simulink model "dynamique_vehicle"  (R2018a)
settings: Solver=ode45  StartTime=0.0  StopTime=10.0  RelTol=1e-3
values from neighbouring files (symbols this model uses):
  Dpitch_h = 1    [Constante.m]
  Droll = hg - (h2+ L2*sin(atan((h1+h2)/L)))    [Constante.m]
  DrollF = DshockF*E1^2    (= 1.44)    [Constante.m]
  DrollR = DshockR*E2^2    (= 1.44)    [Constante.m]
  g = 9.81    [Constante.m]
  Itotx = 1    [Constante.m]
  Itoty = 1    [Constante.m]
  Kpitch_h = 1    [Constante.m]
  KrollF = KspringF*E1^2/2 + KantirollF    (= 1.72)    [Constante.m]
  KrollR = KspringR*E2^2/2 + KantirollR    (= 1.72)    [Constante.m]
  Mtot = 220    [Constante.m]
  Vx0 = 0    [Constante.m]
  Vy0 = 0    [Constante.m]
  Wz0 = 0    [Constante.m]
  X0 = 0    [Constante.m]
  Y0 = 0    [Constante.m]
  yaw0 = 0    [Constante.m]
undefined symbols (not defined in the file or in its folder): Fx1, Fx2, Fx3, Fx4, Fy1, Fy2, Fy3, Fy4
libraries: autolibshareddiff x1
settings Model: Creator=bobau  LastModifiedBy=bobau

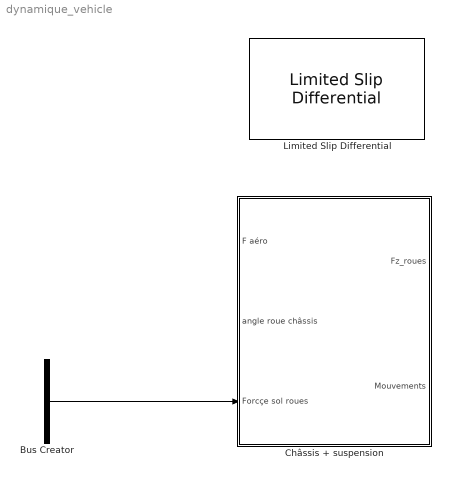
== system dynamique_vehicle ==
  Bus Creator : BusCreator  Inputs=Fy1,Fx1,Fy2,Fx2,Fy3,Fx3,Fy4,Fx4
  Châssis + suspension : Subsystem
  Limited Slip Differential : autolibshareddiff/Limited Slip Differential  shaftSwitchMask=To the left of center-line  Ndiff=4  Jd=.1  bd=1e-3  Jw1=.1  bw1=1e-3  Jw2=.1  bw2=1e-3  omegaw1o=0  omegaw2o=0  couplingType=Pre-loaded ideal clutch  Ndisks=4  Reff=.20  Fc=500  muc=[.16 0.13 0.115 0.11 0.105 0.1025 0.10125]  dw=[0 10 20 40 60 80 100]  Tdw=[-100, -90, -50, -5, 0, 5, 50, 90, 100]  dwT=[-200, -175, -100, - 50, 0, 50, 100, 175, 200]  TTin=[-200 -175 -100 - 50 0 50 100 175 200]  Tin=[-200 -175 -100 - 50 0 50 100 175 200]  tauC=.01  IdealInterpMethod=Linear  IdealExtrapMethod=Clip  TdwInterpMethod=Linear  TdwExtrapMethod=Clip  TTinInterpMethod=Linear  TTinExtrapMethod=Clip  maxAbsSpd=5e3  aMode=2
      settings: SourceProductName=Powertrain Blockset  SourceProductBaseCode=PW
  wires:
  Bus Creator/1 -> Châssis + suspension/3(Forcçe sol roues)

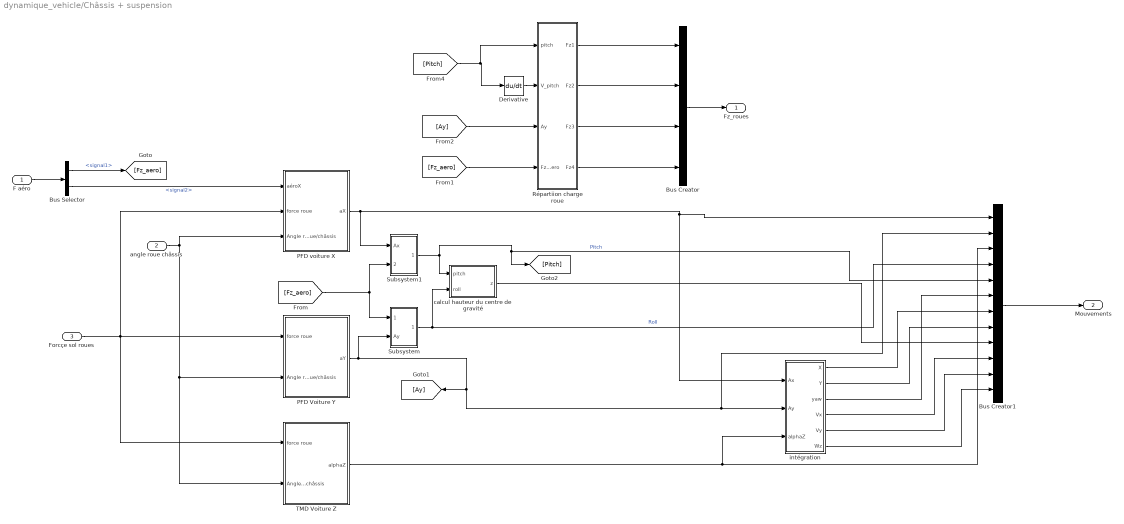
== system dynamique_vehicle/Châssis + suspension ==
  F aéro : Inport
  angle roue châssis : Inport  Port=2
  Forcçe sol roues : Inport  Port=3
  Bus Creator : BusCreator  Inputs=4
  Bus Creator1 : BusCreator  Inputs=12
  Bus Selector : BusSelector  OutputSignals=signal1,signal2
  Derivative : Derivative
  PFD Voiture Y : Subsystem
  PFD voiture X : Subsystem
  Répartiion charge roue : MATLAB Function  TreatAsAtomicUnit=on
  Subsystem : Subsystem
  Subsystem1 : Subsystem
  TMD Voiture Z : Subsystem
  calcul hauteur du centre de gravité : MATLAB Function  TreatAsAtomicUnit=on
  intégration : Subsystem
  Fz_roues : Outport
  Mouvements : Outport  Port=2
  wires:
  Forcçe sol roues/1 -> PFD Voiture Y/1("force roue "), TMD Voiture Z/1("force roue "), PFD voiture X/2("force roue ")
  angle roue châssis/1 -> PFD Voiture Y/2(Angle roue/châssis), TMD Voiture Z/2(Angle roue/châssis), PFD voiture X/3(Angle roue/châssis)
  PFD voiture X/1(aX) -> Bus Creator1/1, intégration/1(Ax), Subsystem1/1(Ax)
  Subsystem/1(Roll) -> calcul hauteur du centre de gravité/2(roll), Bus Creator1/4  "Roll"
  PFD Voiture Y/1(aY) -> Subsystem/2(Ay), Bus Creator1/2, intégration/2(Ay), [Ay]
  Subsystem1/1(Pitch) -> Bus Creator1/5, [Pitch], calcul hauteur du centre de gravité/1(pitch)  "Pitch"
  calcul hauteur du centre de gravité/1(z) -> Bus Creator1/9
  F aéro/1 -> Bus Selector/1
  Bus Selector/2 -> PFD voiture X/1(aéroX)  "<signal2>"
  Bus Selector/1 -> [Fz_aero]  "<signal1>"
  [Fz_aero] -> Subsystem1/2(Fz aéro), Subsystem/1(Fy aéro)
  Derivative/1 -> Répartiion charge roue/2(V_pitch)
  [Fz_aero] -> Répartiion charge roue/4(Fz_aero)
  [Pitch] -> Répartiion charge roue/1(pitch), Derivative/1
  [Ay] -> Répartiion charge roue/3(Ay)
  Répartiion charge roue/1(Fz1) -> Bus Creator/1
  Répartiion charge roue/4(Fz4) -> Bus Creator/4
  Répartiion charge roue/3(Fz3) -> Bus Creator/3
  Répartiion charge roue/2(Fz2) -> Bus Creator/2
  Bus Creator/1 -> Fz_roues/1
  Bus Creator1/1 -> Mouvements/1
  TMD Voiture Z/1(alphaZ) -> Bus Creator1/3, intégration/3(alphaZ)
  intégration/6(Wz) -> Bus Creator1/12
  intégration/5(Vy) -> Bus Creator1/11
  intégration/4(Vx) -> Bus Creator1/10
  intégration/3(yaw) -> Bus Creator1/6
  intégration/2(Y) -> Bus Creator1/8
  intégration/1(X) -> Bus Creator1/7

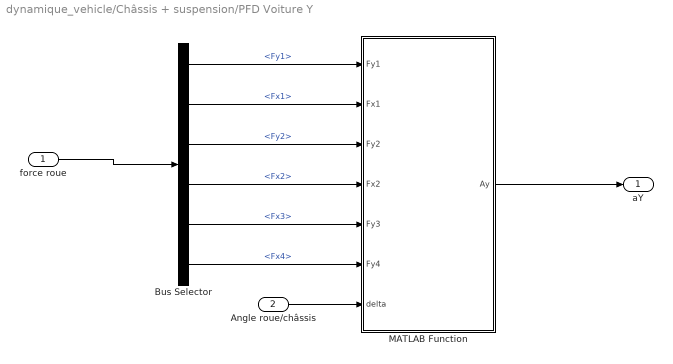
== system dynamique_vehicle/Châssis + suspension/PFD Voiture Y ==
  "force roue " : Inport
  Angle roue/châssis : Inport  Port=2
  Bus Selector : BusSelector  OutputSignals=Fy1,Fx1,Fy2,Fx2,Fx3,Fx4
  MATLAB Function : MATLAB Function  TreatAsAtomicUnit=on
  aY : Outport
  wires:
  Bus Selector/5 -> MATLAB Function/5(Fy3)  "<Fx3>"
  Bus Selector/4 -> MATLAB Function/4(Fx2)  "<Fx2>"
  Bus Selector/3 -> MATLAB Function/3(Fy2)  "<Fy2>"
  Bus Selector/2 -> MATLAB Function/2(Fx1)  "<Fx1>"
  Bus Selector/1 -> MATLAB Function/1(Fy1)  "<Fy1>"
  Bus Selector/6 -> MATLAB Function/6(Fy4)  "<Fx4>"
  Angle roue/châssis/1 -> MATLAB Function/7(delta)
  MATLAB Function/1(Ay) -> aY/1
  "force roue "/1 -> Bus Selector/1

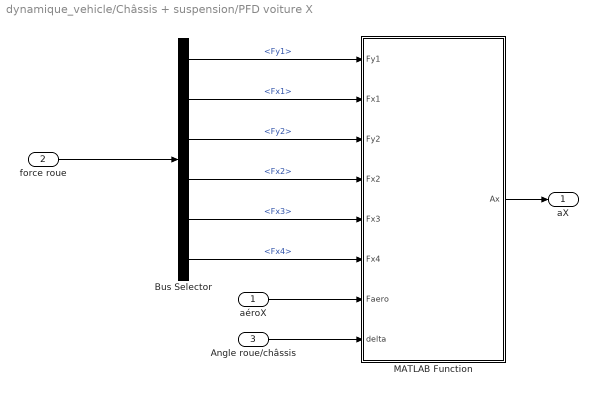
== system dynamique_vehicle/Châssis + suspension/PFD voiture X ==
  aéroX : Inport
  "force roue " : Inport  Port=2
  Angle roue/châssis : Inport  Port=3
  Bus Selector : BusSelector  OutputSignals=Fy1,Fx1,Fy2,Fx2,Fx3,Fx4
  MATLAB Function : MATLAB Function  TreatAsAtomicUnit=on
  aX : Outport
  wires:
  "force roue "/1 -> Bus Selector/1
  MATLAB Function/1(Ax) -> aX/1
  Angle roue/châssis/1 -> MATLAB Function/8(delta)
  Bus Selector/6 -> MATLAB Function/6(Fx4)  "<Fx4>"
  Bus Selector/1 -> MATLAB Function/1(Fy1)  "<Fy1>"
  Bus Selector/2 -> MATLAB Function/2(Fx1)  "<Fx1>"
  Bus Selector/3 -> MATLAB Function/3(Fy2)  "<Fy2>"
  Bus Selector/4 -> MATLAB Function/4(Fx2)  "<Fx2>"
  Bus Selector/5 -> MATLAB Function/5(Fx3)  "<Fx3>"
  aéroX/1 -> MATLAB Function/7(Faero)

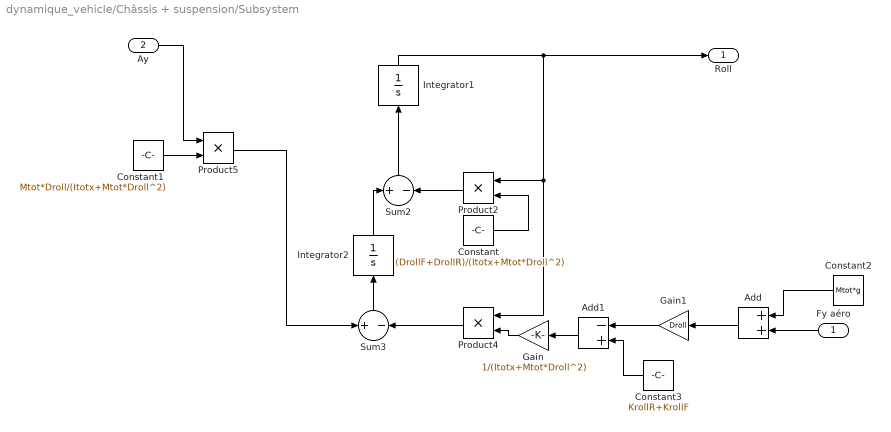
== system dynamique_vehicle/Châssis + suspension/Subsystem ==
  Fy aéro : Inport
  Ay : Inport  Port=2
  Add : Sum
  Add1 : Sum  Inputs=-+
  Constant : Constant  Value=(DrollF+DrollR)/(Itotx+Mtot*Droll^2)
  Constant1 : Constant  Value=Mtot*Droll/(Itotx+Mtot*Droll^2)
  Constant2 : Constant  Value=Mtot*g
  Constant3 : Constant  Value=KrollR+KrollF
  Gain : Gain  Gain=1/(Itotx+Mtot*Droll^2)
  Gain1 : Gain  Gain=Droll
  Integrator1 : Integrator
  Integrator2 : Integrator
  Product2 : Product  SaturateOnIntegerOverflow=on  RndMeth=Zero  InputSameDT=on  OutDataTypeStr=Inherit: Same as first input
  Product4 : Product  SaturateOnIntegerOverflow=on  RndMeth=Zero  InputSameDT=on  OutDataTypeStr=Inherit: Same as first input
  Product5 : Product  SaturateOnIntegerOverflow=on  RndMeth=Zero  InputSameDT=on  OutDataTypeStr=Inherit: Same as first input
  Sum2 : Sum  Inputs=+|-  SaturateOnIntegerOverflow=on  InputSameDT=on  OutDataTypeStr=Inherit: Same as first input
  Sum3 : Sum  Inputs=+|-  SaturateOnIntegerOverflow=on  InputSameDT=on  OutDataTypeStr=Inherit: Same as first input
  Roll : Outport
  wires:
  Ay/1 -> Product5/1
  Product2/1 -> Sum2/2
  Constant/1 -> Product2/2
  Sum3/1 -> Integrator2/1
  Sum2/1 -> Integrator1/1
  Integrator1/1 -> Roll/1, Product2/1, Product4/1
  Gain/1 -> Product4/2
  Product4/1 -> Sum3/2
  Constant3/1 -> Add1/2
  Integrator2/1 -> Sum2/1
  Product5/1 -> Sum3/1
  Constant2/1 -> Add/1
  Add1/1 -> Gain/1
  Constant1/1 -> Product5/2
  Fy aéro/1 -> Add/2
  Gain1/1 -> Add1/1
  Add/1 -> Gain1/1

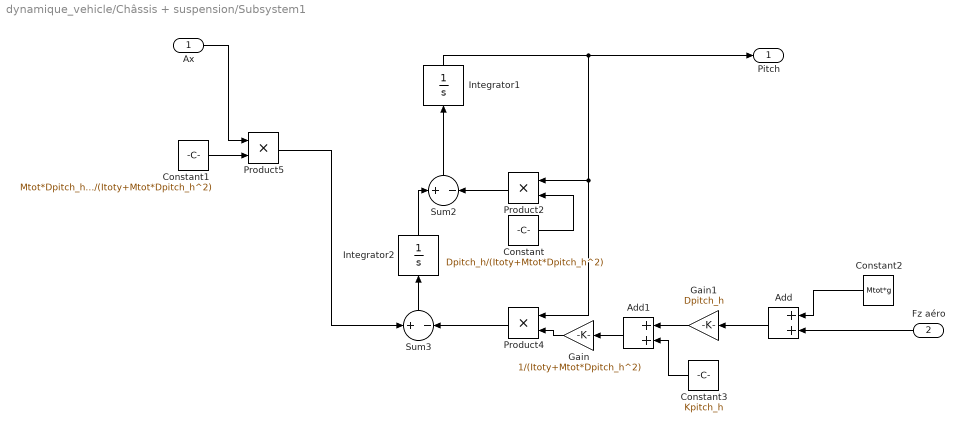
== system dynamique_vehicle/Châssis + suspension/Subsystem1 ==
  Ax : Inport
  Fz aéro : Inport  Port=2
  Add : Sum
  Add1 : Sum
  Constant : Constant  Value=Dpitch_h/(Itoty+Mtot*Dpitch_h^2)
  Constant1 : Constant  Value=Mtot*Dpitch_h/(Itoty+Mtot*Dpitch_h^2)
  Constant2 : Constant  Value=Mtot*g
  Constant3 : Constant  Value=Kpitch_h
  Gain : Gain  Gain=1/(Itoty+Mtot*Dpitch_h^2)
  Gain1 : Gain  Gain=Dpitch_h
  Integrator1 : Integrator
  Integrator2 : Integrator
  Product2 : Product  SaturateOnIntegerOverflow=on  RndMeth=Zero  InputSameDT=on  OutDataTypeStr=Inherit: Same as first input
  Product4 : Product  SaturateOnIntegerOverflow=on  RndMeth=Zero  InputSameDT=on  OutDataTypeStr=Inherit: Same as first input
  Product5 : Product  SaturateOnIntegerOverflow=on  RndMeth=Zero  InputSameDT=on  OutDataTypeStr=Inherit: Same as first input
  Sum2 : Sum  Inputs=+|-  SaturateOnIntegerOverflow=on  InputSameDT=on  OutDataTypeStr=Inherit: Same as first input
  Sum3 : Sum  Inputs=+|-  SaturateOnIntegerOverflow=on  InputSameDT=on  OutDataTypeStr=Inherit: Same as first input
  Pitch : Outport
  wires:
  Fz aéro/1 -> Add/2
  Constant1/1 -> Product5/2
  Add1/1 -> Gain/1
  Constant2/1 -> Add/1
  Product5/1 -> Sum3/1
  Integrator2/1 -> Sum2/1
  Constant3/1 -> Add1/2
  Product4/1 -> Sum3/2
  Gain/1 -> Product4/2
  Integrator1/1 -> Product4/1, Product2/1, Pitch/1
  Sum2/1 -> Integrator1/1
  Sum3/1 -> Integrator2/1
  Constant/1 -> Product2/2
  Product2/1 -> Sum2/2
  Ax/1 -> Product5/1
  Add/1 -> Gain1/1
  Gain1/1 -> Add1/1

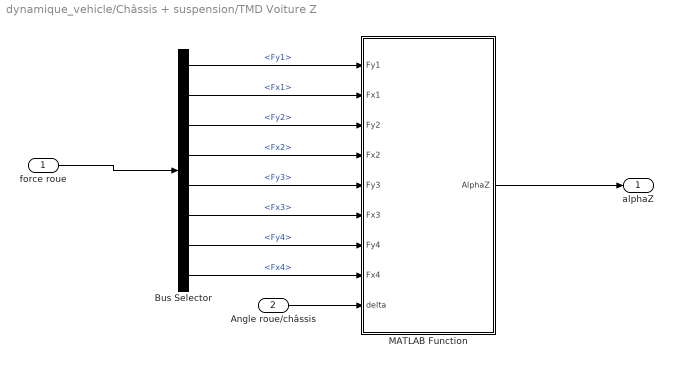
== system dynamique_vehicle/Châssis + suspension/TMD Voiture Z ==
  "force roue " : Inport
  Angle roue/châssis : Inport  Port=2
  Bus Selector : BusSelector  OutputSignals=Fy1,Fx1,Fy2,Fx2,Fy3,Fx3,Fy4,Fx4
  MATLAB Function : MATLAB Function  TreatAsAtomicUnit=on
  alphaZ : Outport
  wires:
  "force roue "/1 -> Bus Selector/1
  MATLAB Function/1(AlphaZ) -> alphaZ/1
  Angle roue/châssis/1 -> MATLAB Function/9(delta)
  Bus Selector/1 -> MATLAB Function/1(Fy1)  "<Fy1>"
  Bus Selector/2 -> MATLAB Function/2(Fx1)  "<Fx1>"
  Bus Selector/3 -> MATLAB Function/3(Fy2)  "<Fy2>"
  Bus Selector/4 -> MATLAB Function/4(Fx2)  "<Fx2>"
  Bus Selector/5 -> MATLAB Function/5(Fy3)  "<Fy3>"
  Bus Selector/6 -> MATLAB Function/6(Fx3)  "<Fx3>"
  Bus Selector/7 -> MATLAB Function/7(Fy4)  "<Fy4>"
  Bus Selector/8 -> MATLAB Function/8(Fx4)  "<Fx4>"

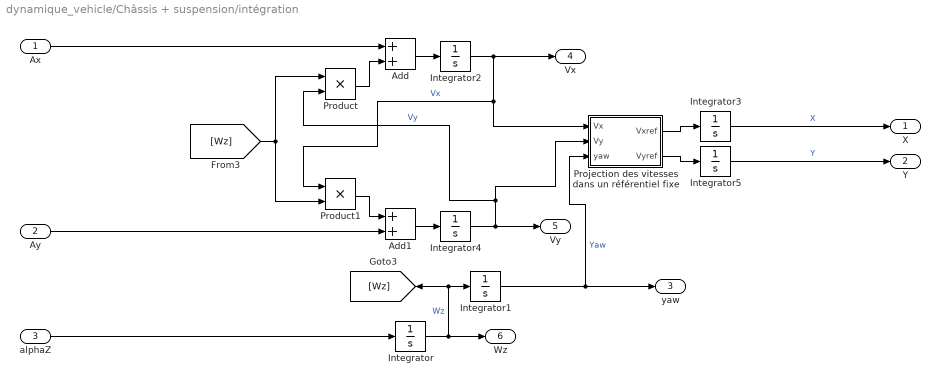
== system dynamique_vehicle/Châssis + suspension/intégration ==
  Ax : Inport
  Ay : Inport  Port=2
  alphaZ : Inport  Port=3
  Add : Sum
  Add1 : Sum
  Integrator : Integrator  InitialCondition=Wz0
  Integrator1 : Integrator  InitialCondition=yaw0
  Integrator2 : Integrator  InitialCondition=Vx0
  Integrator3 : Integrator  InitialCondition=X0
  Integrator4 : Integrator  InitialCondition=Vy0
  Integrator5 : Integrator  InitialCondition=Y0
  Product : Product
  Product1 : Product
  Projection des vitesses dans un référentiel fixe : MATLAB Function  TreatAsAtomicUnit=on
  X : Outport
  Y : Outport  Port=2
  yaw : Outport  Port=3
  Vx : Outport  Port=4
  Vy : Outport  Port=5
  Wz : Outport  Port=6
  wires:
  Integrator/1 -> Wz/1, Integrator1/1, [Wz]  "Wz"
  Add/1 -> Integrator2/1
  Add1/1 -> Integrator4/1
  Integrator4/1 -> Vy/1, Projection des vitesses dans un référentiel fixe/2(Vy), Product/2  "Vy"
  Integrator2/1 -> Vx/1, Projection des vitesses dans un référentiel fixe/1(Vx), Product1/1  "Vx"
  Product/1 -> Add/2
  Product1/1 -> Add1/1
  Integrator3/1 -> X/1  "X"
  [Wz] -> Product1/2, Product/1
  Ay/1 -> Add1/2
  Ax/1 -> Add/1
  alphaZ/1 -> Integrator/1
  Integrator5/1 -> Y/1  "Y"
  Integrator1/1 -> Projection des vitesses dans un référentiel fixe/3(yaw), yaw/1  "Yaw"
  Projection des vitesses dans un référentiel fixe/2(Vyref) -> Integrator5/1
  Projection des vitesses dans un référentiel fixe/1(Vxref) -> Integrator3/1

== matlab function dynamique_vehicle/Châssis + suspension/PFD Voiture Y/MATLAB Function ==
  data: Fy1 input; Fx1 input; Fy2 input; Ay output; Fx2 input; Fy3 input; Fy4 input; delta input
function Ay = PFD_Y(Fy1,Fx1,Fy2,Fx2,Fy3,Fy4,delta)
Ay=(Fy3+Fy4+Faero+(Fy1+Fy2)*cos(delta)+(Fx1+Fx2)*sin(delta))/Mtot;

== matlab function dynamique_vehicle/Châssis + suspension/PFD voiture X/MATLAB Function ==
  data: Fy1 input; Fx1 input; Fy2 input; Ax output; Fx2 input; Fx3 input; Fx4 input; Faero input; delta input
function Ax = fcn(Fy1,Fx1,Fy2,Fx2,Fx3,Fx4,Faero,delta)
Ax=(Fx3+Fx4+Faero+(Fx1+Fx2)*cos(delta)+(Fy1+Fy2)*sin(delta))/Mtot;

== matlab function dynamique_vehicle/Châssis + suspension/TMD Voiture Z/MATLAB Function ==
  data: Fy1 input; Fx1 input; Fy2 input; AlphaZ output; Fx2 input; Fy3 input; Fx3 input; Fy4 input; Fx4 input; delta input
function AlphaZ = TMC_Z(Fy1,Fx1,Fy2,Fx2,Fy3,Fx3,Fy4,Fx4,delta)
AlphaZ = (((Fx1 + Fx2)*sin(delta)+(Fy1 + Fy2)*cos(delta))*L1 -( Fy3 + Fy4)*L2+((Fx2-Fx1)*cos(delta)+(Fy1-Fy2)*sin(delta))*E1/2+(Fx4-Fx3)*E2/2)/Itoty;

== matlab function dynamique_vehicle/Châssis + suspension/calcul hauteur du centre de gravité ==
  data: pitch input; roll input; z output
function z = fcn(pitch, roll)

z = hg + Dpitch_h*(cos(pitch)-1) + Droll*(cos(roll-1));

== matlab function dynamique_vehicle/Châssis + suspension/Répartiion charge roue ==
  data: pitch input; V_pitch input; Fz1 output; Fz2 output; Fz3 output; Fz4 output; Ay input; Fz_aero input
function [Fz1,Fz2,Fz3,Fz4]= fcn(pitch, V_pitch, Ay, Fz_aero)
%la j'avoue j'ai recopié en prenant slope et bank nul (ce sont les
%paramètre d'inclinaisons de la route
DzF = KrollF*Mtot*Droll/E1/(KrollF+KrollR-(Mtot*g+Fz_aero));
DzR = KrollR*Mtot*Droll/E2/(KrollF+KrollR-(Mtot*g+Fz_aero));

Fz1 = (Mtot*g+Fz_aero)/2*L2/(L2+L1)-DzF*Ay-(KspringF/2*L1*tan(pitch)+DshockF*L1*V_pitch)/2;

Fz2 = (Mtot*g+Fz_aero)/2*L2/(L2+L1)+DzF*Ay-(KspringF/2*L1*tan(pitch)+DshockF*L1*V_pitch)/2;

Fz3 = (Mtot*g+Fz_aero)/2*L1/(L2+L1)-DzR*Ay+(KspringR/2*L2*tan(pitch)+DshockR*L2*V_pitch)/2;

Fz4 = (Mtot*g+Fz_aero)/2*L1/(L2+L1)+DzR*Ay+(KspringR/2*L2*tan(pitch)+DshockR*L2*V_pitch)/2;

== matlab function dynamique_vehicle/Châssis + suspension/intégration/Projection des vitesses dans un référentiel fixe ==
  data: Vx input; Vy input; Vxref output; yaw input; Vyref output
function [Vxref,Vyref]= fcn(Vx, Vy, yaw)
Vxref = cos(yaw)*Vx+sin(yaw)*Vy;
Vyref = cos(yaw)*Vy-sin(yaw)*Vx;
